simulink model "passthru_hdl"  (R2021b)
settings: Solver=FixedStepDiscrete  StartTime=0.0  StopTime=SimTime  RelTol=1e-3
values from neighbouring files (symbols this model uses):
  Ts = 1/SIM.fs    [passthru_setup.m]
libraries: hdlsllib x8, xilinxrfsoclib x8, simulink x1
settings Model: Creator=jxperez  LastModifiedBy=brian
settings SolverCC: AlgebraicLoopSolver=TrustRegion
settings DataIOCC: ExternalInput=tx_data  SaveFormat=Array
settings OptimizationCC: BlockReduction=off  ConditionallyExecuteInputs=off  DefaultParameterBehavior=Inlined
settings DebuggingCC: AlgebraicLoopMsg=error  SingleTaskRateTransMsg=error  SFMachineParentedDataDiag=warning
settings HardwareCC: ProdBitPerPointer=32  ProdBitPerSizeT=32  ProdBitPerPtrDiffT=32  ProdLargestAtomicFloat=None  ProdIntDivRoundTo=Undefined  ProdEndianess=Unspecified  ProdWordSize=32  ProdHWDeviceType=ASIC/FPGA->ASIC/FPGA  TargetBitPerLong=64  TargetBitPerPointer=64  TargetBitPerSizeT=64  TargetBitPerPtrDiffT=64  TargetLongLongMode=on  TargetIntDivRoundTo=Zero  TargetEndianess=LittleEndian  TargetWordSize=64  TargetHWDeviceType=Custom Processor->MATLAB Host Computer  ProdEqTarget=off

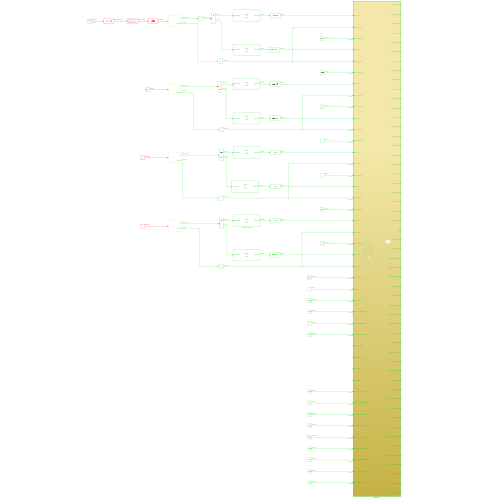
[thumbnail: Simulink's stored preview of the top-level diagram]
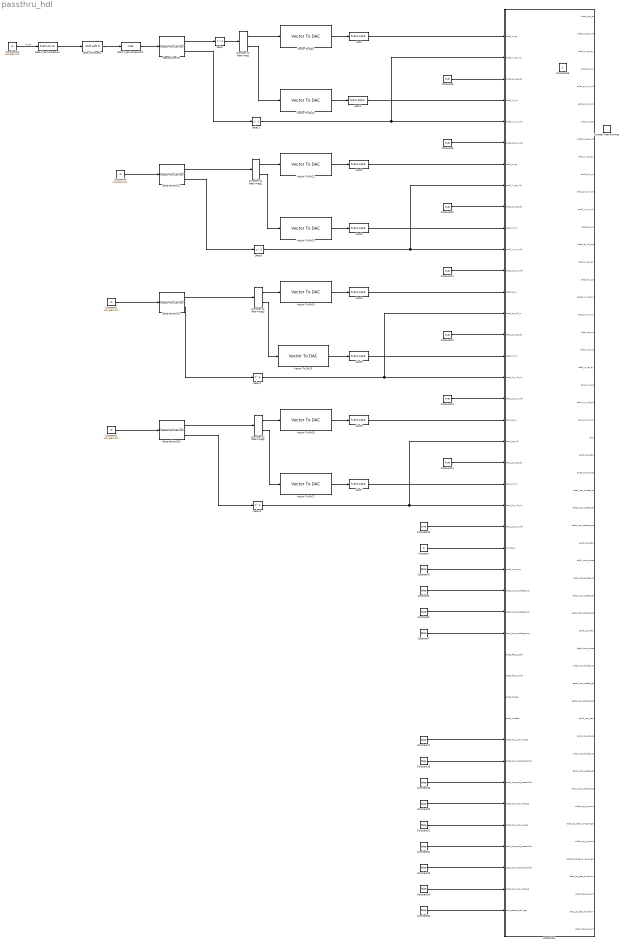
== system passthru_hdl ==
  Cast{,1..7} (8 alike) : DataTypeConversion  OutDataTypeStr=fixdt(1,128,0)
  Complex to Real-Imag{,1..3} (4 alike) : ComplexToRealImag
  Constant : Constant  Value=0  OutDataTypeStr=Inherit: Inherit via back propagation  SampleTime=Ts
  Constant{1..2,4,16} (4 alike) : Constant  Value=complex(0,0)  OutDataTypeStr=int16  SampleTime=Ts/8
  Constant{8..15} (8 alike) : Constant  Value=true  OutDataTypeStr=Inherit: Inherit via back propagation  SampleTime=Ts
  Constant{3,5..7,17..24} (12 alike) : Constant  Value=false  OutDataTypeStr=Inherit: Inherit via back propagation  SampleTime=Ts
  Constant25 : Constant  Value=false  OutDataTypeStr=uint32  SampleTime=Ts
  Data Type Conversion : DataTypeConversion  OutDataTypeStr=fixdt(1,12,11)  SaturateOnIntegerOverflow=on
  Data Type Conversion2 : DataTypeConversion  OutDataTypeStr=int16  SaturateOnIntegerOverflow=on
  Delay{,1..3,5} (5 alike) : Delay  DelayLength=1
  Deserializer1D{,1..3} (4 alike) : hdlsllib/HDL Operations/Deserializer1D  Ratio=8  IdleCycles=0  InitialCondition=0  startIn=off  validIn=off  validOut=on  inputDataDimensions=-1  inputSampleTime=-1  inputSignalType=auto
      settings: SourceProductBaseCode=SL
  PASSTHRU : Subsystem  TreatAsAtomicUnit=on
  Shift Arithmetic : ArithShift  BinPtShiftNumber=14  BitShiftDirection=Left
  Vector To DAC{,1..7} (8 alike) : xilinxrfsoclib/Vector To DAC  INPUT_WL=16  DT_INPUT=0
      settings: SourceProductBaseCode=XILINX_BLOCKSET
  Constant26 : Constant  IOType=siggen
  Counter Free-Running : simulink/Sources/Counter Free-Running  IOType=siggen  NumBits=16  tsamp=-1
  wires:
  Delay/1 -> Complex to Real-Imag/1
  Constant16/1 -> Data Type Conversion/1  "rx_sig"
  Data Type Conversion/1 -> Shift Arithmetic/1
  Deserializer1D/2 -> Delay1/1
  Delay1/1 -> PASSTHRU/2(adc0_in_re_vld), PASSTHRU/5(adc0_in_im_vld)
  Shift Arithmetic/1 -> Data Type Conversion2/1
  Data Type Conversion2/1 -> Deserializer1D/1
  Deserializer1D/1 -> Delay/1
  Constant4/1 -> Deserializer1D1/1
  Complex to Real-Imag/1 -> Vector To DAC/1
  Vector To DAC/1 -> Cast/1
  Cast/1 -> PASSTHRU/1(adc0_in_re)
  Vector To DAC1/1 -> Cast1/1
  Complex to Real-Imag/2 -> Vector To DAC1/1
  Cast1/1 -> PASSTHRU/4(adc0_in_im)
  Vector To DAC2/1 -> Cast2/1
  Vector To DAC3/1 -> Cast3/1
  Deserializer1D1/1 -> Complex to Real-Imag1/1
  Complex to Real-Imag1/1 -> Vector To DAC2/1
  Complex to Real-Imag1/2 -> Vector To DAC3/1
  Cast2/1 -> PASSTHRU/7(adc2_in_re)
  Cast3/1 -> PASSTHRU/10(adc2_in_im)
  Deserializer1D1/2 -> Delay5/1
  Delay5/1 -> PASSTHRU/8(adc2_in_re_vld), PASSTHRU/11(adc2_in_im_vld)
  Delay2/1 -> PASSTHRU/14(dac0_re_vld_in), PASSTHRU/17(dac0_im_vld_in)
  Deserializer1D2/2 -> Delay2/1
  Cast5/1 -> PASSTHRU/16(dac0_im_in)
  Cast4/1 -> PASSTHRU/13(dac0_re_in)
  Complex to Real-Imag2/2 -> Vector To DAC5/1
  Complex to Real-Imag2/1 -> Vector To DAC4/1
  Deserializer1D2/1 -> Complex to Real-Imag2/1
  Vector To DAC5/1 -> Cast5/1
  Vector To DAC4/1 -> Cast4/1
  Constant1/1 -> Deserializer1D2/1
  Constant2/1 -> Deserializer1D3/1
  Vector To DAC6/1 -> Cast6/1
  Vector To DAC7/1 -> Cast7/1
  Deserializer1D3/1 -> Complex to Real-Imag3/1
  Complex to Real-Imag3/1 -> Vector To DAC6/1
  Complex to Real-Imag3/2 -> Vector To DAC7/1
  Cast6/1 -> PASSTHRU/19(dac1_re_in)
  Cast7/1 -> PASSTHRU/22(dac1_im_in)
  Deserializer1D3/2 -> Delay3/1
  Delay3/1 -> PASSTHRU/20(dac1_re_vld), PASSTHRU/23(dac1_im_vld_in)
  Constant/1 -> PASSTHRU/25(switches)
  Constant3/1 -> PASSTHRU/26(adc0_nco_busy)
  Constant5/1 -> PASSTHRU/27(adc2_nco_update_busy)
  Constant6/1 -> PASSTHRU/28(dac0_nco_update_busy)
  Constant7/1 -> PASSTHRU/29(dac1_nco_update_busy)
  Constant8/1 -> PASSTHRU/3(adc0_out_re_rdy)
  Constant9/1 -> PASSTHRU/6(adc0_out_im_rdy)
  Constant10/1 -> PASSTHRU/9(adc2_out_re_rdy)
  Constant11/1 -> PASSTHRU/12(adc2_out_im_rdy)
  Constant12/1 -> PASSTHRU/15(dac0_out_re_rdy)
  Constant13/1 -> PASSTHRU/18(dac0_out_im_rdy)
  Constant14/1 -> PASSTHRU/21(dac1_out_re_rdy)
  Constant15/1 -> PASSTHRU/24(dac1_out_im_rdy)
  Constant17/1 -> PASSTHRU/34(adc0_rts__over_range)
  Constant18/1 -> PASSTHRU/35(adc0_rts_over_threshold1)
  Constant19/1 -> PASSTHRU/36(adc0_rts_over_threshold2)
  Constant20/1 -> PASSTHRU/37(adc0_rts_over_voltage)
  Constant21/1 -> PASSTHRU/38(adc2_rts__over_range)
  Constant22/1 -> PASSTHRU/39(adc2_rts_over_threshold1)
  Constant23/1 -> PASSTHRU/40(adc2_rts_over_threshold2)
  Constant24/1 -> PASSTHRU/41(adc2_rts_over_voltage)
  Constant25/1 -> PASSTHRU/42(adc_capture_ctrl_reg)

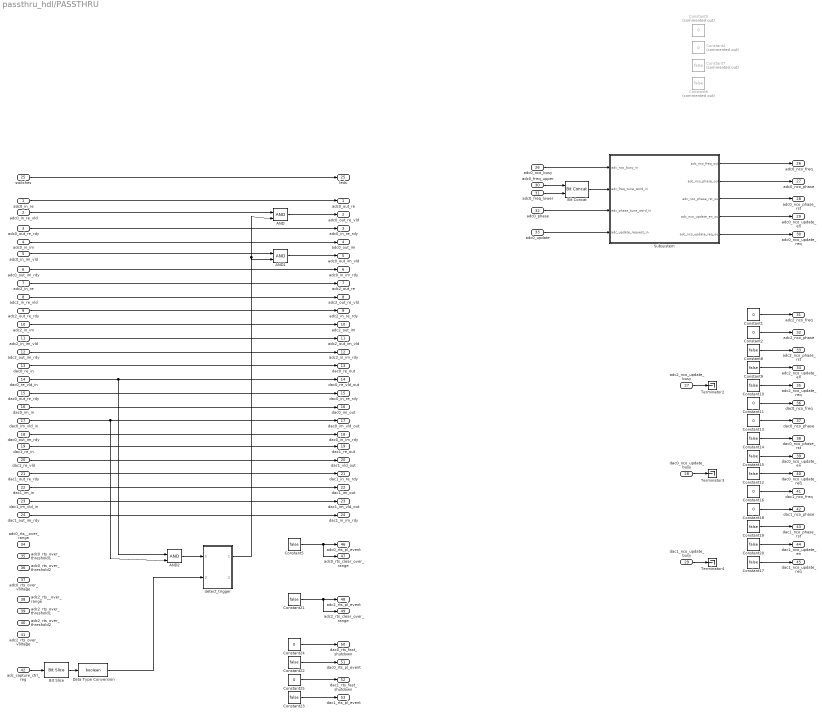
== system passthru_hdl/PASSTHRU ==
  adc0_in_re : Inport
  adc0_in_re_vld : Inport  Port=2
  adc0_out_re_rdy : Inport  Port=3  OutDataTypeStr=boolean
  adc0_in_im : Inport  Port=4
  adc0_in_im_vld : Inport  Port=5
  adc0_out_im_rdy : Inport  Port=6  OutDataTypeStr=boolean
  adc2_in_re : Inport  Port=7
  adc2_in_re_vld : Inport  Port=8  OutDataTypeStr=boolean
  adc2_out_re_rdy : Inport  Port=9  OutDataTypeStr=boolean
  adc2_in_im : Inport  Port=10
  adc2_in_im_vld : Inport  Port=11  OutDataTypeStr=boolean
  adc2_out_im_rdy : Inport  Port=12  OutDataTypeStr=boolean
  dac0_re_in : Inport  Port=13
  dac0_re_vld_in : Inport  Port=14  OutDataTypeStr=boolean
  dac0_out_re_rdy : Inport  Port=15  OutDataTypeStr=boolean
  dac0_im_in : Inport  Port=16
  dac0_im_vld_in : Inport  Port=17  OutDataTypeStr=boolean
  dac0_out_im_rdy : Inport  Port=18  OutDataTypeStr=boolean
  dac1_re_in : Inport  Port=19
  dac1_re_vld : Inport  Port=20
  dac1_out_re_rdy : Inport  Port=21  OutDataTypeStr=boolean
  dac1_im_in : Inport  Port=22
  dac1_im_vld_in : Inport  Port=23
  dac1_out_im_rdy : Inport  Port=24  OutDataTypeStr=boolean
  switches : Inport  Port=25  OutDataTypeStr=fixdt(0,4,0)
  adc0_nco_busy : Inport  Port=26  OutDataTypeStr=boolean
  adc2_nco_update_busy : Inport  Port=27  OutDataTypeStr=boolean
  dac0_nco_update_busy : Inport  Port=28  OutDataTypeStr=boolean
  dac1_nco_update_busy : Inport  Port=29  OutDataTypeStr=boolean
  adc0_freq_upper : Inport  Port=30  OutDataTypeStr=uint32  SampleTime=Ts  LockScale=on
  adc0_freq_lower : Inport  Port=31  OutDataTypeStr=uint32  SampleTime=Ts  LockScale=on
  adc0_phase : Inport  Port=32  OutDataTypeStr=int32  SampleTime=Ts  LockScale=on
  adc0_update : Inport  Port=33  OutMin=0  OutMax=2^6-1  OutDataTypeStr=fixdt(0,6)  SampleTime=Ts  LockScale=on
  adc0_rts__over_range : Inport  Port=34  OutDataTypeStr=boolean
  adc0_rts_over_threshold1 : Inport  Port=35  OutDataTypeStr=boolean
  adc0_rts_over_threshold2 : Inport  Port=36  OutDataTypeStr=boolean
  adc0_rts_over_voltage : Inport  Port=37  OutDataTypeStr=boolean
  adc2_rts__over_range : Inport  Port=38  OutDataTypeStr=boolean
  adc2_rts_over_threshold1 : Inport  Port=39  OutDataTypeStr=boolean
  adc2_rts_over_threshold2 : Inport  Port=40  OutDataTypeStr=boolean
  adc2_rts_over_voltage : Inport  Port=41  OutDataTypeStr=boolean
  adc_capture_ctrl_reg : Inport  Port=42  OutMin=0  OutMax=2^6-1  OutDataTypeStr=uint32  SampleTime=Ts  LockScale=on
  AND : Logic  IconShape=distinctive  AllPortsSameDT=off  OutDataTypeStr=boolean
  AND1 : Logic  IconShape=distinctive  AllPortsSameDT=off  OutDataTypeStr=boolean
  AND2 : Logic  IconShape=distinctive  AllPortsSameDT=off  OutDataTypeStr=boolean
  Bit Concat : hdlsllib/Logic and Bit Operations/Bit Concat  numInputs=2
  Bit Slice : hdlsllib/Logic and Bit Operations/Bit Slice  lidx=31  ridx=31
      settings: SourceProductBaseCode=SL
  Constant1 : Constant  Value=0  OutDataTypeStr=fixdt(1,48,47)  SampleTime=Ts
  Constant{8,10,12,14,17,19} (6 alike) : Constant  Value=false  OutDataTypeStr=boolean  SampleTime=Ts
  Constant11 : Constant  Value=0  OutDataTypeStr=fixdt(1,48,47)  SampleTime=Ts
  Constant13 : Constant  Value=0  OutDataTypeStr=fixdt(1,18,17)  SampleTime=Ts
  Constant15 : Constant  Value=false  OutDataTypeStr=fixdt(0,6,0)  SampleTime=Ts
  Constant16 : Constant  Value=0  OutDataTypeStr=fixdt(1,48,47)  SampleTime=Ts
  Constant18 : Constant  Value=0  OutDataTypeStr=fixdt(1,18,17)  SampleTime=Ts
  Constant2 : Constant  Value=0  OutDataTypeStr=fixdt(1,18,17)  SampleTime=Ts
  Constant20 : Constant  Value=false  OutDataTypeStr=fixdt(0,6,0)  SampleTime=Ts
  Constant{5,21..23} (4 alike) : Constant  Value=false  OutDataTypeStr=Inherit: Inherit via back propagation  SampleTime=Ts
  Constant24 : Constant  Value=0  OutMin=0  OutDataTypeStr=fixdt(0,3)  SampleTime=Ts
  Constant25 : Constant  Value=0  OutMin=0  OutDataTypeStr=fixdt(0,3)  SampleTime=Ts
  Constant3 : Constant  Commented=on  Value=0  OutDataTypeStr=fixdt(1,48,47)  SampleTime=Ts
  Constant4 : Constant  Commented=on  Value=0  OutDataTypeStr=fixdt(1,18,17)  SampleTime=Ts
  Constant6 : Constant  Commented=on  Value=false  OutDataTypeStr=fixdt(0,6,0)  SampleTime=Ts
  Constant7 : Constant  Commented=on  Value=false  OutDataTypeStr=boolean  SampleTime=Ts
  Constant9 : Constant  Value=false  OutDataTypeStr=fixdt(0,6,0)  SampleTime=Ts
  Data Type Conversion : DataTypeConversion  OutDataTypeStr=boolean
  Subsystem : Subsystem
  Terminator2 : Terminator
  Terminator3 : Terminator
  Terminator4 : Terminator
  detect_trigger : Subsystem  ReferencedSubsystem=set_reset_ff_2
  adc0_out_re : Outport
  adc0_out_re_vld : Outport  Port=2
  adc0_in_re_rdy : Outport  Port=3
  adc0_out_im : Outport  Port=4
  adc0_out_im_vld : Outport  Port=5
  adc0_in_im_rdy : Outport  Port=6
  adc2_out_re : Outport  Port=7
  adc2_out_re_vld : Outport  Port=8
  adc2_in_re_rdy : Outport  Port=9
  adc2_out_im : Outport  Port=10
  adc2_out_im_vld : Outport  Port=11
  adc2_in_im_rdy : Outport  Port=12
  dac0_re_out : Outport  Port=13
  dac0_re_vld_out : Outport  Port=14
  dac0_in_re_rdy : Outport  Port=15
  dac0_im_out : Outport  Port=16
  dac0_im_vld_out : Outport  Port=17
  dac0_in_im_rdy : Outport  Port=18
  dac1_re_out : Outport  Port=19
  dac1_vld_out : Outport  Port=20
  dac1_in_re_rdy : Outport  Port=21
  dac1_im_out : Outport  Port=22
  dac1_im_vld_out : Outport  Port=23
  dac1_in_im_rdy : Outport  Port=24
  leds : Outport  Port=25
  adc0_nco_freq : Outport  Port=26
  adc0_nco_phase : Outport  Port=27
  adc0_nco_phase_rst : Outport  Port=28
  adc0_nco_update_en : Outport  Port=29
  adc0_nco_update_req : Outport  Port=30
  adc2_nco_freq : Outport  Port=31
  adc2_nco_phase : Outport  Port=32
  adc2_nco_phase_rst : Outport  Port=33
  adc2_nco_update_en : Outport  Port=34
  adc2_nco_update_req : Outport  Port=35
  dac0_nco_freq : Outport  Port=36
  dac0_nco_phase : Outport  Port=37
  dac0_nco_phase_rst : Outport  Port=38
  dac0_nco_update_en : Outport  Port=39
  dac0_nco_update_req : Outport  Port=40
  dac1_nco_freq : Outport  Port=41
  dac1_nco_phase : Outport  Port=42
  dac1_nco_phase_rst : Outport  Port=43
  dac1_nco_update_en : Outport  Port=44
  dac1_nco_update_req : Outport  Port=45
  adc0_rts_pl_event : Outport  Port=46  OutDataTypeStr=boolean
  adc0_rts_clear_over_range : Outport  Port=47  OutDataTypeStr=boolean
  adc2_rts_pl_event : Outport  Port=48  OutDataTypeStr=boolean
  adc2_rts_clear_over_range : Outport  Port=49  OutDataTypeStr=boolean
  dac0_rts_fast_shutdown : Outport  Port=50  OutMin=0  OutDataTypeStr=fixdt(0,3)
  dac0_rts_pl_event : Outport  Port=51  OutDataTypeStr=boolean
  dac1_rts_fast_shutdown : Outport  Port=52  OutMin=0  OutDataTypeStr=fixdt(0,3)
  dac1_rts_pl_event : Outport  Port=53  OutDataTypeStr=boolean
  wires:
  adc0_in_im/1 -> adc0_out_im/1
  switches/1 -> leds/1
  adc0_in_re/1 -> adc0_out_re/1
  adc2_in_re/1 -> adc2_out_re/1
  adc2_in_im/1 -> adc2_out_im/1
  adc2_in_re_vld/1 -> adc2_out_re_vld/1
  adc2_in_im_vld/1 -> adc2_out_im_vld/1
  dac0_re_in/1 -> dac0_re_out/1
  dac0_re_vld_in/1 -> AND2/1, dac0_re_vld_out/1
  dac0_im_in/1 -> dac0_im_out/1
  dac0_im_vld_in/1 -> AND2/2, dac0_im_vld_out/1
  dac1_re_in/1 -> dac1_re_out/1
  dac1_re_vld/1 -> dac1_vld_out/1
  dac1_im_in/1 -> dac1_im_out/1
  dac1_im_vld_in/1 -> dac1_im_vld_out/1
  adc2_nco_update_busy/1 -> Terminator2/1
  Constant10/1 -> adc2_nco_update_req/1
  Constant9/1 -> adc2_nco_update_en/1
  Constant8/1 -> adc2_nco_phase_rst/1
  Constant2/1 -> adc2_nco_phase/1
  Constant1/1 -> adc2_nco_freq/1
  Constant11/1 -> dac0_nco_freq/1
  Constant13/1 -> dac0_nco_phase/1
  Constant14/1 -> dac0_nco_phase_rst/1
  Constant15/1 -> dac0_nco_update_en/1
  Constant12/1 -> dac0_nco_update_req/1
  dac0_nco_update_busy/1 -> Terminator3/1
  dac1_nco_update_busy/1 -> Terminator4/1
  Constant17/1 -> dac1_nco_update_req/1
  Constant20/1 -> dac1_nco_update_en/1
  Constant19/1 -> dac1_nco_phase_rst/1
  Constant18/1 -> dac1_nco_phase/1
  Constant16/1 -> dac1_nco_freq/1
  adc0_out_re_rdy/1 -> adc0_in_re_rdy/1
  adc0_out_im_rdy/1 -> adc0_in_im_rdy/1
  adc2_out_re_rdy/1 -> adc2_in_re_rdy/1
  adc2_out_im_rdy/1 -> adc2_in_im_rdy/1
  dac0_out_re_rdy/1 -> dac0_in_re_rdy/1
  dac0_out_im_rdy/1 -> dac0_in_im_rdy/1
  dac1_out_re_rdy/1 -> dac1_in_re_rdy/1
  dac1_out_im_rdy/1 -> dac1_in_im_rdy/1
  adc0_nco_busy/1 -> Subsystem/1(adc_nco_busy_in)
  adc0_phase/1 -> Subsystem/3(adc_phase_tune_word_in)
  adc0_update/1 -> Subsystem/4(adc_update_request_in)
  Subsystem/1(adc_nco_freq_out) -> adc0_nco_freq/1
  Subsystem/2(adc_nco_phase_out) -> adc0_nco_phase/1
  Subsystem/3(adc_nco_phase_rst_out) -> adc0_nco_phase_rst/1
  Subsystem/4(adc_nco_update_en_out) -> adc0_nco_update_en/1
  Subsystem/5(adc_nco_update_req_out) -> adc0_nco_update_req/1
  adc0_freq_upper/1 -> Bit Concat/1
  adc0_freq_lower/1 -> Bit Concat/2
  Bit Concat/1 -> Subsystem/2(adc_freq_tune_word_in)
  Constant5/1 -> adc0_rts_clear_over_range/1, adc0_rts_pl_event/1
  Constant21/1 -> adc2_rts_clear_over_range/1, adc2_rts_pl_event/1
  Constant22/1 -> dac0_rts_pl_event/1
  Constant23/1 -> dac1_rts_pl_event/1
  Constant24/1 -> dac0_rts_fast_shutdown/1
  Constant25/1 -> dac1_rts_fast_shutdown/1
  AND/1 -> adc0_out_re_vld/1
  adc0_in_re_vld/1 -> AND/1
  detect_trigger/1 -> AND1/2, AND/2
  AND1/1 -> adc0_out_im_vld/1
  adc0_in_im_vld/1 -> AND1/1
  Bit Slice/1 -> Data Type Conversion/1
  adc_capture_ctrl_reg/1 -> Bit Slice/1
  Data Type Conversion/1 -> detect_trigger/2
  AND2/1 -> detect_trigger/1

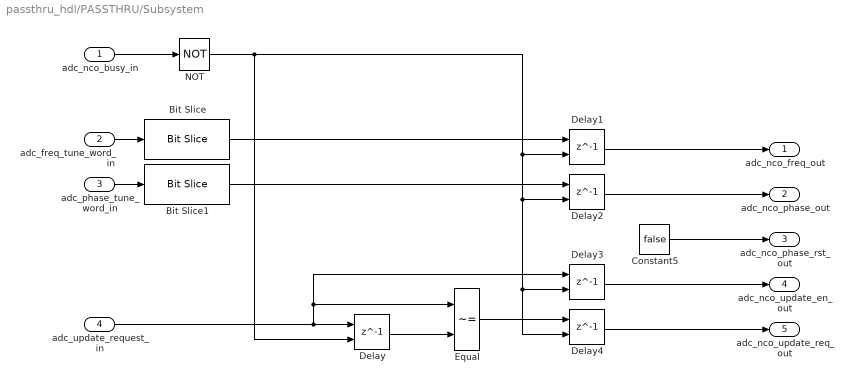
== system passthru_hdl/PASSTHRU/Subsystem ==
  adc_nco_busy_in : Inport
  adc_freq_tune_word_in : Inport  Port=2
  adc_phase_tune_word_in : Inport  Port=3
  adc_update_request_in : Inport  Port=4
  Bit Slice : hdlsllib/Logic and Bit Operations/Bit Slice  lidx=63  ridx=16
      settings: SourceProductBaseCode=SL
  Bit Slice1 : hdlsllib/Logic and Bit Operations/Bit Slice  lidx=31  ridx=32-18
      settings: SourceProductBaseCode=SL
  Constant5 : Constant  Value=false  OutDataTypeStr=boolean  SampleTime=Ts
  Delay{,1..4} (5 alike) : Delay  DelayLength=1  ShowEnablePort=on  SampleTime=Ts
      settings: InputPortMap=u0,e6
  Equal : RelationalOperator  Operator=~=  OutDataTypeStr=boolean  RndMeth=Simplest
  NOT : Logic  Operator=NOT  IconShape=distinctive  AllPortsSameDT=off  OutDataTypeStr=boolean
  adc_nco_freq_out : Outport
  adc_nco_phase_out : Outport  Port=2
  adc_nco_phase_rst_out : Outport  Port=3
  adc_nco_update_en_out : Outport  Port=4
  adc_nco_update_req_out : Outport  Port=5
  wires:
  Bit Slice/1 -> Delay1/1
  Equal/1 -> Delay4/1
  adc_update_request_in/1 -> Delay3/1, Equal/1, Delay/1
  Delay/1 -> Equal/2
  Delay3/1 -> adc_nco_update_en_out/1
  Delay1/1 -> adc_nco_freq_out/1
  Delay4/1 -> adc_nco_update_req_out/1
  Bit Slice1/1 -> Delay2/1
  adc_nco_busy_in/1 -> NOT/1
  adc_freq_tune_word_in/1 -> Bit Slice/1
  Constant5/1 -> adc_nco_phase_rst_out/1
  Delay2/1 -> adc_nco_phase_out/1
  NOT/1 -> Delay4/2, Delay3/2, Delay2/2, Delay1/2, Delay/2
  adc_phase_tune_word_in/1 -> Bit Slice1/1
